simulink model "D1_simuprueba"  (R2018a)
settings: Solver=VariableStepAuto  StartTime=0.0  StopTime=100  RelTol=1e-3
undefined symbols (not defined in the file or in its folder): dQ, dS2, nQ, nS2
settings Model: Creator=quich  LastModifiedBy=glori

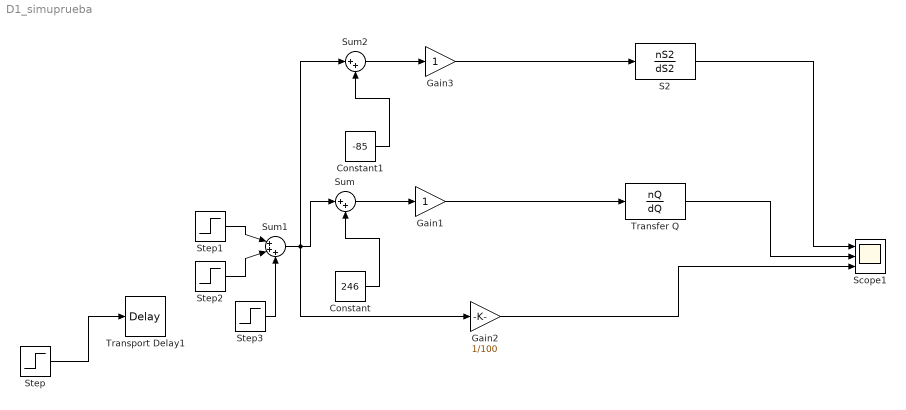
== system D1_simuprueba ==
  Constant : Constant  Value=246  SampleTime=0.055
  Constant1 : Constant  Value=-85  SampleTime=0.055
  Gain1 : Gain
  Gain2 : Gain  Gain=1/100
  Gain3 : Gain
  S2 : TransferFcn  Numerator=nS2  Denominator=dS2
  Scope1 : Scope  NumInputPorts=3
  Step : Step  Time=193  SampleTime=0
  Step1 : Step  Time=35  Before=193  After=314  SampleTime=0
  Step2 : Step  Time=55  After=120  SampleTime=0
  Step3 : Step  Time=70  After=97  SampleTime=0
  Sum : Sum  Inputs=|++
  Sum1 : Sum  Inputs=|+++
  Sum2 : Sum  Inputs=|++
  Transfer Q : TransferFcn  Numerator=nQ  Denominator=dQ
  Transport Delay1 : TransportDelay  DelayTime=5
  wires:
  Step/1 -> Transport Delay1/1
  Transfer Q/1 -> Scope1/2
  Gain2/1 -> Scope1/3
  Sum/1 -> Gain1/1
  Constant/1 -> Sum/2
  Gain1/1 -> Transfer Q/1
  Step1/1 -> Sum1/1
  Sum1/1 -> Sum2/1, Gain2/1, Sum/1
  Step2/1 -> Sum1/2
  Step3/1 -> Sum1/3
  Sum2/1 -> Gain3/1
  Constant1/1 -> Sum2/2
  Gain3/1 -> S2/1
  S2/1 -> Scope1/1
